simulink model "fileTest"  (R2017b)
settings: Solver=FixedStepAuto  StartTime=0.0  StopTime=inf  FixedStep=.001  RelTol=1e-3  EnableMultiTasking=on
libraries: simulink x1
settings Model: SimulationMode=external  Creator=dskaputa  LastModifiedBy=dskaputa
settings SolverCC: PositivePriorityOrder=on
settings OptimizationCC: PassReuseOutputArgsAs=Individual arguments  MaxStackSize=64
settings DebuggingCC: ParameterTunabilityLossMsg=error
settings HardwareCC: ProdBitPerPointer=32  ProdBitPerSizeT=32  ProdBitPerPtrDiffT=32  ProdLargestAtomicInteger=Long  ProdLargestAtomicFloat=Double  ProdWordSize=32  ProdHWDeviceType=ARM Compatible->ARM Cortex
settings SFSimCC: MATLABDynamicMemAlloc=off
settings RTWCC: SystemTargetFile=ert.tlc  HardwareBoard=ZedBoard  TemplateMakefile=ert_default_tmf  GenerateReport=on  Toolchain=Xilinx Software Development Kit (SDK)  IncludeHyperlinkInReport=on  LaunchReport=on  GenerateTraceInfo=on  GenerateTraceReport=on  GenerateTraceReportSl=on  GenerateTraceReportSf=on  GenerateTraceReportEml=on
settings CodeAppCC: ForceParamTrailComments=on  IgnoreCustomStorageClasses=off  OperatorAnnotations=on  SimulinkDataObjDesc=on  SFDataObjDesc=on  MATLABFcnDesc=on  InsertBlockDesc=on  StateflowObjectComments=on  MATLABSourceComments=on
settings ERTTargetCC: SupportNonInlinedSFcns=on

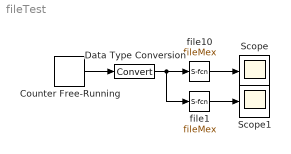
== system fileTest ==
  Counter Free-Running : simulink/Sources/Counter Free-Running  NumBits=16  tsamp=-1
  Data Type Conversion : DataTypeConversion
  Scope : Scope
  Scope1 : Scope
  file1 : S-Function  FunctionName=fileMex  Parameters=param1  SFunctionDeploymentMode=off  EnableBusSupport=off  mask{param1=2}
      mask prompts: param1 "File Index"
      mask Display: image('D:\snickDrone\mexFiles\file\fileImage.png');
  file10 : S-Function  FunctionName=fileMex  Parameters=param1  SFunctionDeploymentMode=off  EnableBusSupport=off  mask{param1=1}
      mask prompts: param1 "File Index"
      mask Display: image('D:\snickDrone\mexFiles\file\fileImage.png');
  wires:
  file10/1 -> Scope/1
  Counter Free-Running/1 -> Data Type Conversion/1
  Data Type Conversion/1 -> file1/1, file10/1
  file1/1 -> Scope1/1
